simulink model "quizq1"  (R2013b)
settings: Solver=ode4  StartTime=0.0  StopTime=0.04  FixedStep=0.0001  RelTol=1e-3
settings Model: Creator=Zeerak Nadeem Wyne  LastModifiedBy=Zeerak Nadeem Wyne

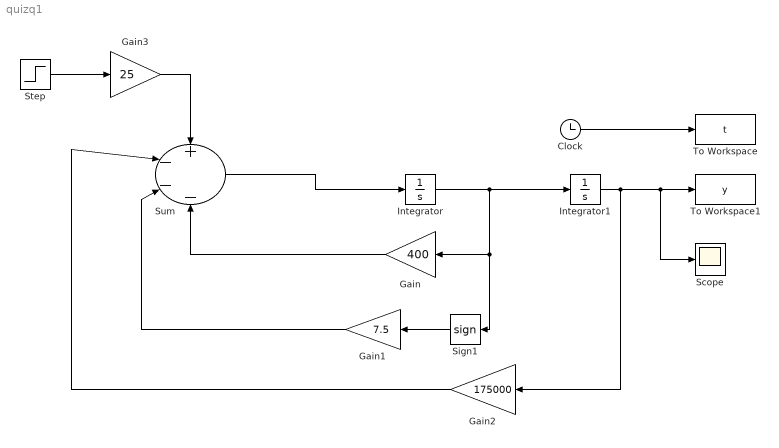
== system quizq1 ==
  Clock : Clock
  Gain : Gain  Gain=400
  Gain1 : Gain  Gain=7.5
  Gain2 : Gain  Gain=175000
  Gain3 : Gain  Gain=25
  Integrator : Integrator
  Integrator1 : Integrator  InitialCondition=0.000473
  Scope : Scope
      settings: YMin=0.44935  YMax=0.49665
  Sign1 : Signum
  Step : Step  Time=0  After=12  SampleTime=0.0001
  Sum : Sum  Inputs=+---
  To Workspace : ToWorkspace  VariableName=t  SampleTime=-1
  To Workspace1 : ToWorkspace  VariableName=y  SampleTime=-1
  wires:
  Integrator/1 -> Sign1/1, Gain/1, Integrator1/1
  Gain/1 -> Sum/4
  Integrator1/1 -> Scope/1, To Workspace1/1, Gain2/1
  Gain2/1 -> Sum/2
  Step/1 -> Gain3/1
  Clock/1 -> To Workspace/1
  Gain1/1 -> Sum/3
  Sum/1 -> Integrator/1
  Gain3/1 -> Sum/1
  Sign1/1 -> Gain1/1
